simulink subsystem "pulse"  (R2022b)
settings: Solver=VariableStepAuto  StartTime=0.0  StopTime=10.0  RelTol=1e-3
Description:
  | Copyright (c) 2023, Alexei Evsenin, evsenin@gmail.com
settings Model: Creator=evsenin  LastModifiedBy=evsenin
settings DebuggingCC: UnconnectedInputMsg=warning  UnconnectedOutputMsg=warning  UnconnectedLineMsg=warning
settings ModelReferenceCC: EnableRefExpFcnMdlSchedulingChecks=on
settings RTWCC: DLArmComputeVersion=19.05

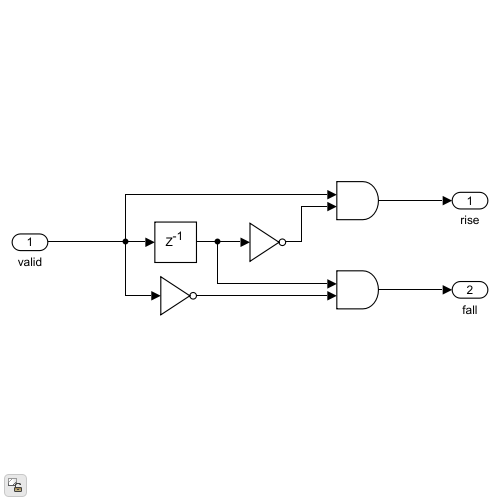
[thumbnail: Simulink's stored preview of the top-level diagram]
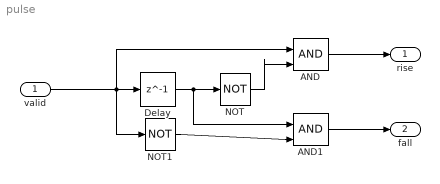
== system pulse ==
  valid : Inport
  AND : Logic  IconShape=distinctive  AllPortsSameDT=off  OutDataTypeStr=boolean
  AND1 : Logic  IconShape=distinctive  AllPortsSameDT=off  OutDataTypeStr=boolean
  Delay : Delay  DelayLength=1
  NOT : Logic  Operator=NOT  IconShape=distinctive  AllPortsSameDT=off  OutDataTypeStr=boolean
  NOT1 : Logic  Operator=NOT  IconShape=distinctive  AllPortsSameDT=off  OutDataTypeStr=boolean
  rise : Outport
  fall : Outport  Port=2
  wires:
  NOT/1 -> AND/2
  valid/1 -> Delay/1, NOT1/1, AND/1
  AND/1 -> rise/1
  Delay/1 -> NOT/1, AND1/1
  NOT1/1 -> AND1/2
  AND1/1 -> fall/1
